simulink model "z1_airport"  (R2017b)
settings: Solver=FixedStepDiscrete  StartTime=0.0  StopTime=0  RelTol=1e-3
libraries: CPOiS_SourcesSinks x9, CPOiS_HistogramOperations x3
settings Model: Creator=alis  LastModifiedBy=alis

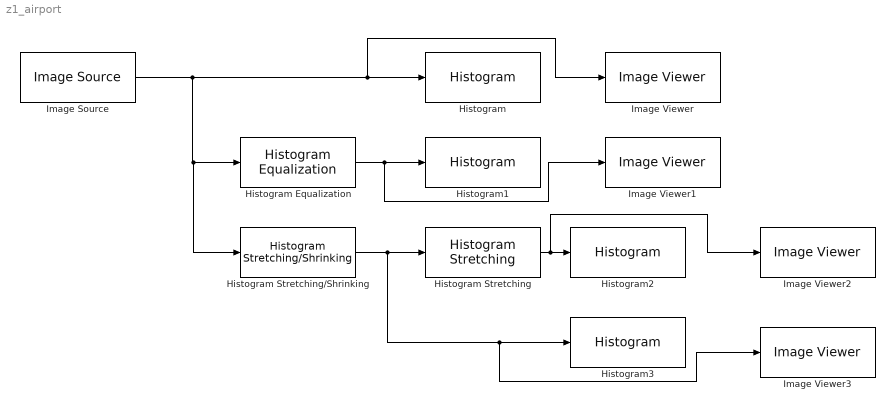
== system z1_airport ==
  Histogram{,1..3} (4 alike) : CPOiS_SourcesSinks/Histogram
      settings: SourceProductName=CPOiS - Digital image and signal processing
  Histogram Stretching/Shrinking : CPOiS_HistogramOperations/Histogram Stretching//Shrinking  minimum=0  maximum=122
      settings: SourceProductName=CPOiS - Digital image and signal processing
  Histogram Equalization : CPOiS_HistogramOperations/Histogram Equalization
      settings: SourceProductName=CPOiS - Digital image and signal processing
  Histogram Stretching : CPOiS_HistogramOperations/Histogram Stretching
      settings: SourceProductName=CPOiS - Digital image and signal processing
  Image Source : CPOiS_SourcesSinks/Image Source  FileSelection=airport.png
      settings: SourceProductName=CPOiS - Digital image and signal processing
  Image Viewer{,1..3} (4 alike) : CPOiS_SourcesSinks/Image Viewer
      settings: SourceProductName=CPOiS - Digital image and signal processing
  wires:
  Image Source/1 -> Histogram Stretching/Shrinking/1, Histogram Equalization/1, Image Viewer/1, Histogram/1
  Histogram Equalization/1 -> Image Viewer1/1, Histogram1/1
  Histogram Stretching/1 -> Image Viewer2/1, Histogram2/1
  Histogram Stretching/Shrinking/1 -> Image Viewer3/1, Histogram3/1, Histogram Stretching/1
